simulink model "EXPT_7_6"  (R2019a)
settings: Solver=VariableStepAuto  StartTime=0.0  StopTime=10.0  RelTol=1e-3
undefined symbols (not defined in the file or in its folder): strel
libraries: visionmorphops x4, visionconversions x4, visionsources x1
settings Model: Creator=91977  LastModifiedBy=91977

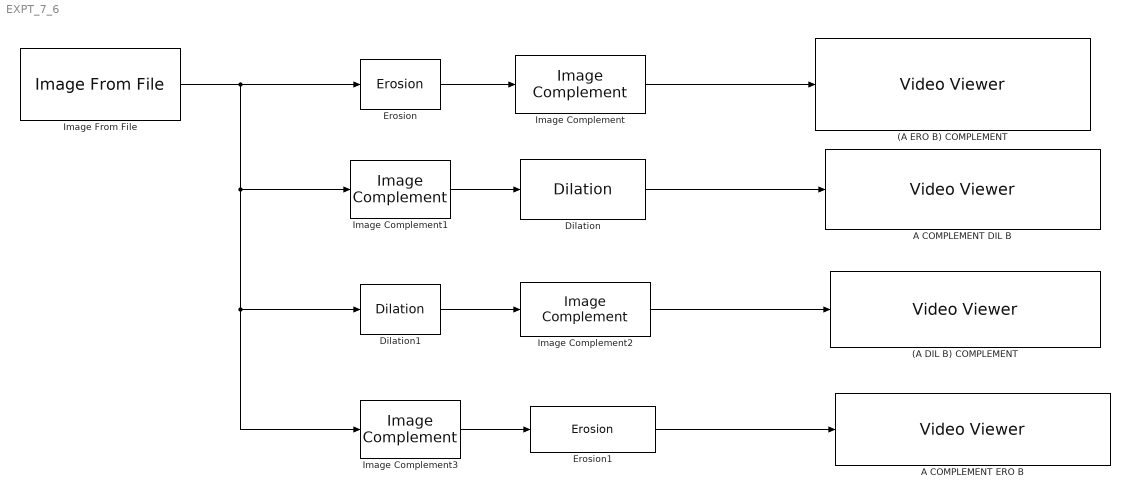
== system EXPT_7_6 ==
  (A DIL B) COMPLEMENT : VideoViewer  FigPos=[160.2 678 417.6 304]
  (A ERO B) COMPLEMENT : VideoViewer  FigPos=[559 583 418 304]
  A COMPLEMENT DIL B : VideoViewer  FigPos=[495.4 872.4 417.6 304]
  A COMPLEMENT ERO B : VideoViewer  FigPos=[945 641.2 417.6 304]
  Dilation : visionmorphops/Dilation  nhoodsrc=Specify via dialog  strel=[1 1; 1 1]
      settings: SourceProductName=Computer Vision Toolbox  SourceProductBaseCode=VP
  Dilation1 : visionmorphops/Dilation  nhoodsrc=Specify via dialog  strel=[1 1; 1 1]
      settings: SourceProductName=Computer Vision Toolbox  SourceProductBaseCode=VP
  Erosion : visionmorphops/Erosion  nhoodsrc=Specify via dialog  strel=strel('square',4)
      settings: SourceProductName=Computer Vision Toolbox  SourceProductBaseCode=VP
  Erosion1 : visionmorphops/Erosion  nhoodsrc=Specify via dialog  strel=strel('square',4)
      settings: SourceProductName=Computer Vision Toolbox  SourceProductBaseCode=VP
  Image Complement{,1..3} (4 alike) : visionconversions/Image Complement
      settings: SourceProductName=Computer Vision Toolbox  SourceProductBaseCode=VP
  Image From File : visionsources/Image From File  Tag=vipblks_nd  FileName=circles.png  Ts=inf  imagePorts=One multidimensional signal  OutPortLabels=R|G|B  ImageDataType=Inherit from input image  sdImageDataType=uint(8)  Signed=on  WordLength=16  FractionLengthMode=User-defined  FractionLength=15
      settings: SourceProductName=Computer Vision Toolbox
  wires:
  Image From File/1 -> Image Complement1/1, Dilation1/1, Image Complement3/1, Erosion/1
  Erosion/1 -> Image Complement/1
  Image Complement/1 -> (A ERO B) COMPLEMENT/1
  Image Complement1/1 -> Dilation/1
  Dilation/1 -> A COMPLEMENT DIL B/1
  Dilation1/1 -> Image Complement2/1
  Image Complement2/1 -> (A DIL B) COMPLEMENT/1
  Image Complement3/1 -> Erosion1/1
  Erosion1/1 -> A COMPLEMENT ERO B/1
